simulink model "SimpleHandModelSim"  (Simulink 7.9)
settings: Solver=ode3  StartTime=0.0  StopTime=tstop  FixedStep=ts  RelTol=1e-3
undefined symbols (not defined in the file or in its folder): Bv, F_grav, HII, L, Lc, m, ml, q0, qd0
libraries: planmant x1
settings Model: Creator=Tadej  LastModifiedBy=Tadej
settings HardwareCC: TargetIntDivRoundTo=Zero  TargetEndianess=LittleEndian  TargetHWDeviceType=MATLAB Host  ProdEqTarget=off
settings RTWCC: SystemTargetFile=rtwsfcn.tlc  TemplateMakefile=rtwsfcn_default_tmf  Description=S-Function Target  ProcessScript=rtwsfcn_make_rtw_hook  RTWCompilerOptimization=On
settings STFCustomTargetCC: CodeReplacementLibrary=ANSI_C  ModelReferenceCompliant=off  CompOptLevelCompliant=on  GeneratePreprocessorConditionals=Disable all  SystemTargetFile=rtwsfcn.tlc
settings CustomProperty: Value=on

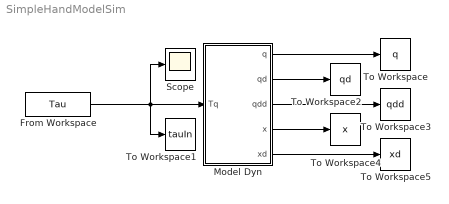
== system SimpleHandModelSim ==
  From Workspace : FromWorkspace  VariableName=Tau  SampleTime=0  Interpolate=off  OutputAfterFinalValue=Holding final value
  Model Dyn : Subsystem  mask(Dynamic model){L=L, Lc=Lc, m=m, ml=ml, HII=HII, Bv=Bv, F_grav=F_grav, q0=q0, qd0=qd0}
      mask prompts: L "Link Lengths [L]:"; Lc "Mass Centerpoints [Lc]:"; m "Link Masses [m]:"; ml "Load Mass [ml]:"; HII "Link Inertias [II]:"; Bv "Viscouse Friction Coeficient. [Bv]:"; F_grav "Gravity Gain [F_grav]:"; q0 "Initial Joit Positions [q0]:"; qd0 "Initial Joit Velocities [qd0]:"
      mask help: Dynamic model of the manipulator
      mask init:
      | nj=length(L);mj=length(kinmodel(q0,L));
      mask Display: disp('Dyn')
  Scope : Scope
  To Workspace : ToWorkspace  VariableName=q  SampleTime=-1  SaveFormat=Structure With Time
  To Workspace1 : ToWorkspace  VariableName=tauIn  SampleTime=-1  SaveFormat=Structure With Time
  To Workspace2 : ToWorkspace  VariableName=qd  SampleTime=-1  SaveFormat=Structure With Time
  To Workspace3 : ToWorkspace  VariableName=qdd  SampleTime=-1  SaveFormat=Structure With Time
  To Workspace4 : ToWorkspace  VariableName=x  SampleTime=-1  SaveFormat=Structure With Time
  To Workspace5 : ToWorkspace  VariableName=xd  SampleTime=-1  SaveFormat=Structure With Time
  wires:
  From Workspace/1 -> Model Dyn/1(Tq), Scope/1, To Workspace1/1
  Model Dyn/1(q) -> To Workspace/1
  Model Dyn/2(qd) -> To Workspace2/1
  Model Dyn/3(qdd) -> To Workspace3/1
  Model Dyn/4(x) -> To Workspace4/1
  Model Dyn/5(xd) -> To Workspace5/1

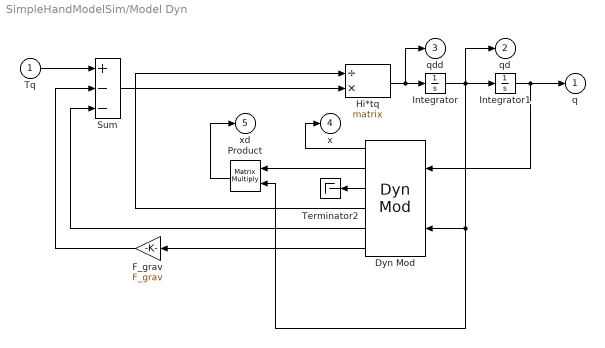
== system SimpleHandModelSim/Model Dyn ==
  Tq : Inport
  Dyn Mod : planmant/Model/Dyn Mod  L=L  Lc=Lc  m=m  ml=ml  HII=HII  Bv=Bv
  F_grav : Gain  Gain=F_grav  SaturateOnIntegerOverflow=on  OutDataTypeStr=Inherit: Same as input  ParamDataTypeStr=Inherit: Same as input
  Hi*tq : Product  Inputs=/*  Multiplication=Matrix(*)  SaturateOnIntegerOverflow=on  InputSameDT=on  OutDataTypeStr=Inherit: Same as first input
  Integrator : Integrator  InitialCondition=qd0
  Integrator1 : Integrator  InitialCondition=q0
  Product : Product  Multiplication=Matrix(*)  RndMeth=Zero
  Sum : Sum  Inputs=+--  SaturateOnIntegerOverflow=on  InputSameDT=on  OutDataTypeStr=Inherit: Same as first input
  Terminator2 : Terminator
  q : Outport  InitialOutput=0
  qd : Outport  Port=2  InitialOutput=0
  qdd : Outport  Port=3  InitialOutput=0
  x : Outport  Port=4  InitialOutput=0
  xd : Outport  Port=5  InitialOutput=0
  wires:
  Tq/1 -> Sum/1
  Dyn Mod/4 -> Hi*tq/1
  Dyn Mod/5 -> Sum/3
  Integrator1/1 -> q/1, Dyn Mod/1
  Integrator/1 -> Integrator1/1, qd/1, Dyn Mod/2, Product/2
  Sum/1 -> Hi*tq/2
  Hi*tq/1 -> Integrator/1, qdd/1
  Dyn Mod/1 -> x/1
  Dyn Mod/2 -> Product/1
  Dyn Mod/3 -> Terminator2/1
  Dyn Mod/6 -> F_grav/1
  F_grav/1 -> Sum/2
  Product/1 -> xd/1
